simulink model "data_valid_example"  (R2020a)
settings: Solver=FixedStepDiscrete  StartTime=0.0  StopTime=600  RelTol=1e-3
undefined symbols (not defined in the file or in its folder): filter_coeff, filter_input, max_gap, NumBits1, NumBits2, Slope1, Slope2
libraries: simulink x3, hdlsllib x3, dspsrcs4 x2
settings Model: DataTypeOverride=Off  Creator=cchung  LastModifiedBy=cchung
settings DataIOCC: SaveOutput=off  SaveTime=off
settings OptimizationCC: BlockReduction=off  ConditionallyExecuteInputs=off  DefaultParameterBehavior=Inlined
settings DebuggingCC: AlgebraicLoopMsg=error  SingleTaskRateTransMsg=error
settings HardwareCC: ProdBitPerPointer=32  ProdBitPerSizeT=32  ProdBitPerPtrDiffT=32  ProdLargestAtomicFloat=None  ProdIntDivRoundTo=Undefined  ProdEndianess=Unspecified  ProdWordSize=32  ProdHWDeviceType=ASIC/FPGA->ASIC/FPGA  TargetBitPerPointer=64  TargetBitPerSizeT=64  TargetBitPerPtrDiffT=64  TargetLongLongMode=on  TargetIntDivRoundTo=Zero  TargetEndianess=LittleEndian  TargetWordSize=64  TargetHWDeviceType=Custom Processor->MATLAB Host Computer  ProdEqTarget=off

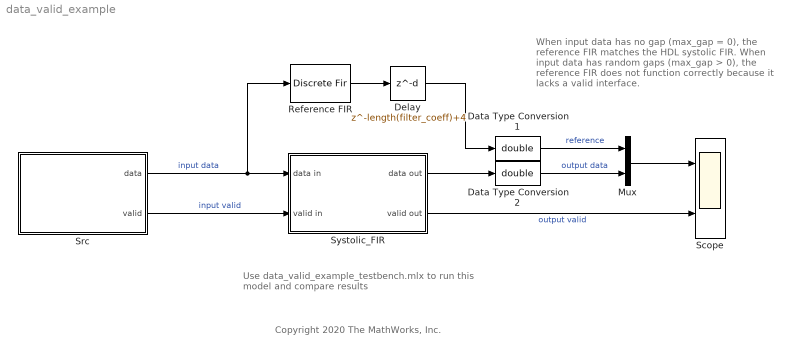
== system data_valid_example ==
  note: Use data_valid_example_testbench.mlx
      | to run this model and compare results
  note: When input data has no gap (max_gap = 0),
      | the reference FIR matches the HDL systolic FIR.
      |
      | When input data has random gaps (max_gap > 0),
      | the reference FIR does not function correctly
      | because it lacks a valid interface.
  note: Copyright 2020 The MathWorks, Inc.
  Data Type Conversion1 : DataTypeConversion  OutDataTypeStr=double
  Data Type Conversion2 : DataTypeConversion  OutDataTypeStr=double
  Delay : Delay  DelayLength=length(filter_coeff)+4
  Mux : Mux  Inputs=2
  Reference FIR : DiscreteFir  Coefficients=filter_coeff
  Scope : Scope  NumInputPorts=2
  Src : Subsystem  mask(Irregular data source){src=filter_input, Ts=1, nsamps=1, min_gap=0, max_gap=max_gap, invalid_src=cast(-1,'like',filter_input)}
      mask prompts: src "Signal:"; Ts "Sample time:"; nsamps "Samples per frame:"; min_gap "Minimum gap (>=0):"; max_gap "Maximum gap (>=0):"; invalid_src "Signal during invalid gap:"
      mask help:
      | Insert irregular gaps between valid data samples. The Signal from Workspace block from DSP System Toolbox is used to stream data specified in 'Signal'. Values specified in 'Signal during invalid gap' is repeated during gap, and when Signal runs out.
      |
      | Sample time Ts is the period of a single sample. e.g. Ts = 1 at 2 samples per frame results in a frame rate of 2.
      |
      | Data is periodic when max gap == min gap; when both are 0, data is always valid (until 'Signal' runs out).
      mask init:
      | if min_gap < 0
      |     error('Minimum gap must be >= 0')
      | end
      | if max_gap < 0
      |     error('Maximum gap must be >= 0')
      | end
      | if min_gap > max_gap
      |     error('Minimum gap must be <= maximum gap')
      | end
      mask TypeOptions Ts:
      | Valid Src/Signal From
      | Workspace/Ts | Invalid Src/Signal From
      | Workspace/Ts
      mask TypeOptions nsamps:
      | Valid Src/Signal From
      | Workspace/nsamps | Invalid Src/Signal From
      | Workspace/nsamps
      mask DialogControl ParameterGroupVar Prompt: Signal Parameters
      mask DialogControl Container3 Prompt: Gap Parameters
      mask Display:
      | s = sprintf('\n\n%d Sample/Frame\n',nsamps);
      | 
      | if min_gap == max_gap
      |     if max_gap == 0
      |         fprintf('Streaming Source%s',s);
      |     else
      |         fprintf('Periodic Source%sEvery %d Cycles',s,max_gap+1);
      |     end
      | else
      |     fprintf('Irregular Source%sEvery %d-%d Cycles',s,min_gap+1,max_gap+1);
      | end
  Systolic_FIR : Subsystem  mask(Systolic FIR Example){coe=filter_coeff}
      mask prompts: coe "Coefficients"
      mask help: This example uses for-each subsystem to cascade taps in a systolic FIR filter.
      mask init:
      | clen = numel(coe);
      mask Display: fprintf('%d-tap Systolic\nFIR Filter',clen);
  wires:
  Src/2(valid) -> Systolic_FIR/2(valid in)  "input valid"
  Src/1(data) -> Reference FIR/1, Systolic_FIR/1(data in)  "input data"
  Data Type Conversion2/1 -> Mux/2  "output data"
  Systolic_FIR/2(valid out) -> Scope/2  "output valid"
  Reference FIR/1 -> Delay/1
  Data Type Conversion1/1 -> Mux/1  "reference"
  Mux/1 -> Scope/1
  Delay/1 -> Data Type Conversion1/1
  Systolic_FIR/1(data out) -> Data Type Conversion2/1

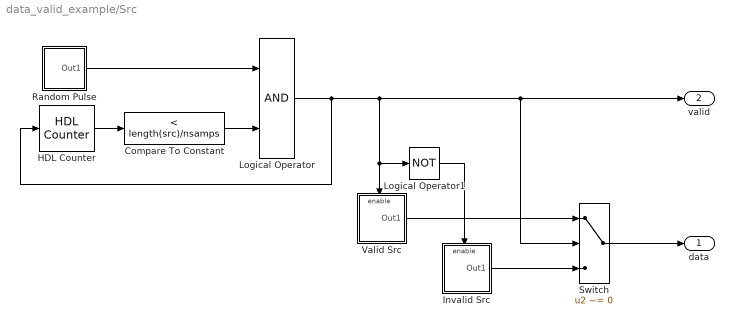
== system data_valid_example/Src ==
  Compare To Constant : simulink/Logic and Bit Operations/Compare To Constant  relop=<  const=length(src)/nsamps  OutDataTypeStr=boolean
  HDL Counter : hdlsllib/Sources/HDL Counter  CountType=Free running  CountInit=0  CountStep=1  CountMax=10  CountFromType=Initial value  CountFrom=0  CountResetPort=off  CountLoadPort=off  CountEnbPort=on  CountDirPort=off  CountDataType=Unsigned  CountWordLen=32  CountFracLen=0  CountSampTime=1
  Invalid Src : Subsystem
  Logical Operator : Logic  AllPortsSameDT=off  OutDataTypeStr=boolean
  Logical Operator1 : Logic  Operator=NOT  AllPortsSameDT=off  OutDataTypeStr=boolean
  Random Pulse : Subsystem
  Switch : Switch  Criteria=u2 ~= 0
  Valid Src : Subsystem
  data : Outport  VectorParamsAs1DForOutWhenUnconnected=off
  valid : Outport  Port=2  VectorParamsAs1DForOutWhenUnconnected=off
  wires:
  Compare To Constant/1 -> Logical Operator/2
  HDL Counter/1 -> Compare To Constant/1
  Logical Operator/1 -> Logical Operator1/1, Valid Src/Enable, Switch/2, valid/1, HDL Counter/1
  Valid Src/1(Out1) -> Switch/1
  Random Pulse/1(Out1) -> Logical Operator/1
  Invalid Src/1(Out1) -> Switch/3
  Switch/1 -> data/1
  Logical Operator1/1 -> Invalid Src/Enable

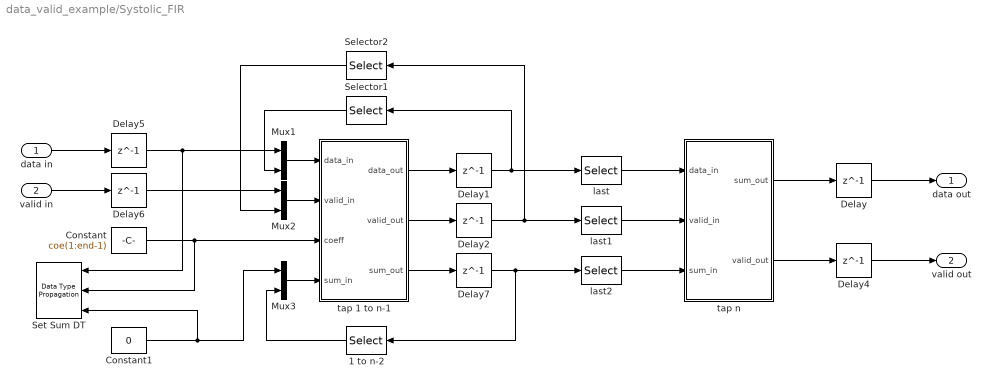
== system data_valid_example/Systolic_FIR ==
  data in : Inport
  valid in : Inport  Port=2
  1 to n-2 : Selector  InputPortWidth=clen-1  IndexOptions=Index vector (dialog)  Indices=1:clen-2  OutputSizes=1
  Constant : Constant  Value=coe(1:end-1)  SampleTime=-1
  Constant1 : Constant  Value=0  OutDataTypeStr=Inherit: Inherit via back propagation  SampleTime=-1
  Delay{,1..2,4..7} (7 alike) : Delay  DelayLength=1
  Mux1 : Mux  Inputs=2
  Mux2 : Mux  Inputs=2
  Mux3 : Mux  Inputs=2
  Selector1 : Selector  InputPortWidth=clen-1  IndexOptions=Index vector (dialog)  Indices=1:clen-2  OutputSizes=1
  Selector2 : Selector  InputPortWidth=clen-1  IndexOptions=Index vector (dialog)  Indices=1:clen-2  OutputSizes=1
  Set Sum DT : simulink/Signal Attributes/Data Type Propagation  PropDataType=fixdt(1, 16)  IfRefDouble=double  IfRefSingle=single  IsSigned=IsSigned1  NumBitsBase=NumBits1+NumBits2  NumBitsMult=1  NumBitsAdd=nextpow2(clen)  NumBitsAllowFinal=1:128  PropScaling=2^-10  ValuesUsedBestPrec=[5 -7]  SlopeBase=Slope1*Slope2  SlopeMult=1  SlopeAdd=0  BiasBase=Bias1  BiasMult=1  BiasAdd=0
      settings: SourceProductBaseCode=SL
  last : Selector  InputPortWidth=clen-1  IndexOptions=Index vector (dialog)  Indices=clen-1  OutputSizes=1
  last1 : Selector  InputPortWidth=clen-1  IndexOptions=Index vector (dialog)  Indices=clen-1  OutputSizes=1
  last2 : Selector  InputPortWidth=clen-1  IndexOptions=Index vector (dialog)  Indices=clen-1  OutputSizes=1
  tap 1 to n-1 : Subsystem  TreatAsAtomicUnit=on
  tap n : Subsystem
  data out : Outport  VectorParamsAs1DForOutWhenUnconnected=off
  valid out : Outport  Port=2  VectorParamsAs1DForOutWhenUnconnected=off
  wires:
  data in/1 -> Delay5/1
  Constant/1 -> Set Sum DT/2, tap 1 to n-1/3(coeff)
  Mux1/1 -> tap 1 to n-1/1(data_in)
  Mux2/1 -> tap 1 to n-1/2(valid_in)
  tap 1 to n-1/1(data_out) -> Delay1/1
  tap 1 to n-1/2(valid_out) -> Delay2/1
  Delay5/1 -> Mux1/1, Set Sum DT/1
  Delay6/1 -> Mux2/1
  Selector2/1 -> Mux2/2
  Selector1/1 -> Mux1/2
  Delay1/1 -> Selector1/1, last/1
  Delay2/1 -> last1/1, Selector2/1
  valid in/1 -> Delay6/1
  Delay4/1 -> valid out/1
  Delay/1 -> data out/1
  tap 1 to n-1/3(sum_out) -> Delay7/1
  Delay7/1 -> last2/1, 1 to n-2/1
  last1/1 -> tap n/2(valid_in)
  last/1 -> tap n/1(data_in)
  last2/1 -> tap n/3(sum_in)
  tap n/1(sum_out) -> Delay/1
  tap n/2(valid_out) -> Delay4/1
  Mux3/1 -> tap 1 to n-1/4(sum_in)
  1 to n-2/1 -> Mux3/2
  Constant1/1 -> Mux3/1, Set Sum DT/3

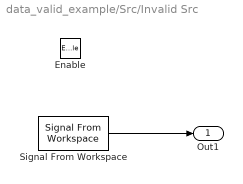
== system data_valid_example/Src/Invalid Src ==
  Enable : EnablePort
  Signal From Workspace : dspsrcs4/Signal From Workspace  X=invalid_src  Ts=Ts  nsamps=nsamps  OutputAfterFinalValue=Cyclic repetition  ignoreOrWarnInputAndFrameLengths=off  OutputFrames=off
  Out1 : Outport  VectorParamsAs1DForOutWhenUnconnected=off
  wires:
  Signal From Workspace/1 -> Out1/1

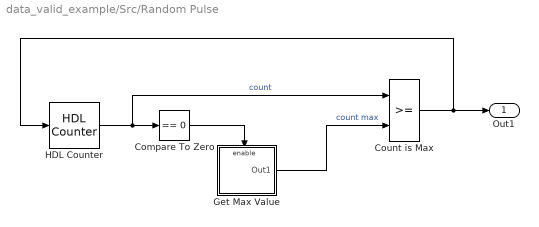
== system data_valid_example/Src/Random Pulse ==
  Compare To Zero : simulink/Logic and Bit Operations/Compare To Zero  relop===  OutDataTypeStr=boolean
  Count is Max : RelationalOperator  OutDataTypeStr=boolean  RndMeth=Nearest
  Get Max Value : Subsystem
  HDL Counter : hdlsllib/Sources/HDL Counter  CountType=Free running  CountInit=0  CountStep=1  CountMax=25  CountFromType=Initial value  CountFrom=0  CountResetPort=on  CountLoadPort=off  CountEnbPort=off  CountDirPort=off  CountDataType=Unsigned  CountWordLen=8  CountFracLen=0  CountSampTime=1
  Out1 : Outport  VectorParamsAs1DForOutWhenUnconnected=off
  wires:
  Count is Max/1 -> Out1/1, HDL Counter/1
  Compare To Zero/1 -> Get Max Value/Enable
  HDL Counter/1 -> Count is Max/1, Compare To Zero/1  "count"
  Get Max Value/1(Out1) -> Count is Max/2  "count max"

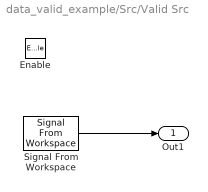
== system data_valid_example/Src/Valid Src ==
  Enable : EnablePort
  Signal From Workspace : dspsrcs4/Signal From Workspace  X=src  Ts=Ts  nsamps=nsamps  OutputAfterFinalValue=Setting to zero  ignoreOrWarnInputAndFrameLengths=off  OutputFrames=off
  Out1 : Outport  VectorParamsAs1DForOutWhenUnconnected=off
  wires:
  Signal From Workspace/1 -> Out1/1

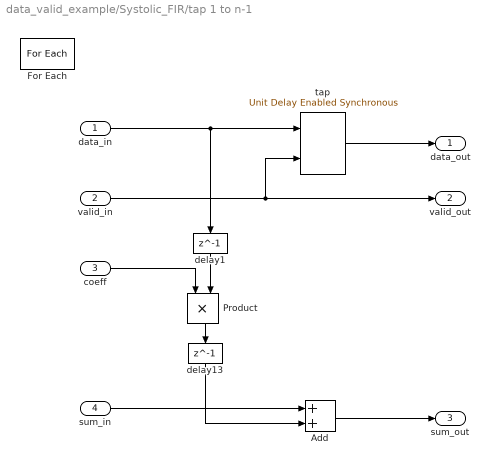
== system data_valid_example/Systolic_FIR/tap 1 to n-1 ==
  data_in : Inport  Partition=on  PartitionDimension=1  PartitionWidth=1  PartitionOffset=0
  valid_in : Inport  Port=2  Partition=on  PartitionDimension=1  PartitionWidth=1  PartitionOffset=0
  coeff : Inport  Port=3  Partition=on  PartitionDimension=1  PartitionWidth=1  PartitionOffset=0
  sum_in : Inport  Port=4  Partition=on  PartitionDimension=1  PartitionWidth=1  PartitionOffset=0
  Add : Sum  OutDataTypeStr=Inherit: Same as accumulator
  For Each : ForEach  DisableCoverage=on
  Product : Product
  delay1 : Delay  DelayLength=1  InitialCondition=0
  delay13 : Delay  DelayLength=1  InitialCondition=0
  tap : hdlsllib/Discrete/Unit Delay Enabled Synchronous  InitialCondition=0.0  SampleTime=-1
      settings: SourceProductBaseCode=SL
  data_out : Outport  ConcatenationDimension=1  VectorParamsAs1DForOutWhenUnconnected=off
  valid_out : Outport  Port=2  ConcatenationDimension=1  VectorParamsAs1DForOutWhenUnconnected=off
  sum_out : Outport  Port=3  ConcatenationDimension=1  VectorParamsAs1DForOutWhenUnconnected=off
  wires:
  coeff/1 -> Product/1
  tap/1 -> data_out/1
  valid_in/1 -> valid_out/1, tap/2
  data_in/1 -> delay1/1, tap/1
  Product/1 -> delay13/1
  delay13/1 -> Add/2
  sum_in/1 -> Add/1
  Add/1 -> sum_out/1
  delay1/1 -> Product/2

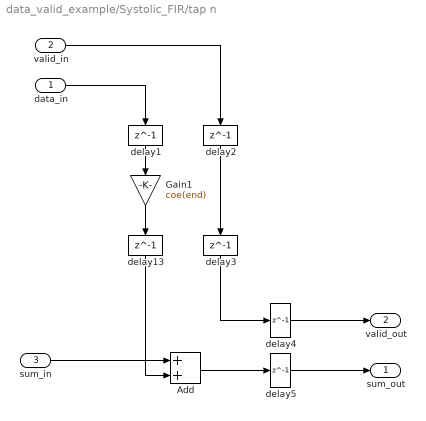
== system data_valid_example/Systolic_FIR/tap n ==
  data_in : Inport
  valid_in : Inport  Port=2
  sum_in : Inport  Port=3
  Add : Sum  OutDataTypeStr=Inherit: Same as accumulator
  Gain1 : Gain  Gain=coe(end)  ParamDataTypeStr=Inherit: Inherit from 'Gain'
  delay{1..5,13} (6 alike) : Delay  DelayLength=1  InitialCondition=0
  sum_out : Outport  VectorParamsAs1DForOutWhenUnconnected=off
  valid_out : Outport  Port=2  VectorParamsAs1DForOutWhenUnconnected=off
  wires:
  valid_in/1 -> delay2/1
  data_in/1 -> delay1/1
  delay13/1 -> Add/2
  delay1/1 -> Gain1/1
  Gain1/1 -> delay13/1
  delay2/1 -> delay3/1
  delay3/1 -> delay4/1
  delay4/1 -> valid_out/1
  delay5/1 -> sum_out/1
  Add/1 -> delay5/1
  sum_in/1 -> Add/1

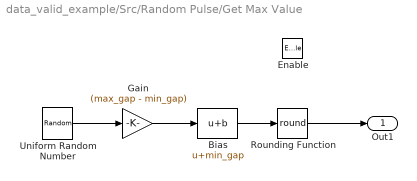
== system data_valid_example/Src/Random Pulse/Get Max Value ==
  Enable : EnablePort
  Bias : Bias  Bias=min_gap
  Gain : Gain  Gain=(max_gap - min_gap)
  Rounding Function : Rounding  Operator=round
  Uniform Random Number : UniformRandomNumber  Minimum=0  Seed=randi([0 100],1)  SampleTime=Ts*nsamps
  Out1 : Outport  VectorParamsAs1DForOutWhenUnconnected=off
  wires:
  Rounding Function/1 -> Out1/1
  Uniform Random Number/1 -> Gain/1
  Gain/1 -> Bias/1
  Bias/1 -> Rounding Function/1
